simulink model "model"  (R2021a)
settings: Solver=ode4  StartTime=0.0  StopTime=sim_time  FixedStep=0.001  RelTol=1e-3
values from neighbouring files (symbols this model uses):
  ABS_ON = 0    [initialization.m]    (also in result_analysis.m = 1)
  Af = 2.36    [initialization.m]
  battery_capacity = 58*3.6*10^6    (= 208800000)    [initialization.m]
  battery_limit = 99    [initialization.m]
  brake_start = 10    [initialization.m]    (also in result_analysis.m)
  brakes = 1    [initialization.m]    (also in result_analysis.m)
  Cm = 310    [initialization.m]
  Cx = 0.27    [initialization.m]
  EBD_ON = 0    [initialization.m]    (also in result_analysis.m = 1)
  eta = 0.90    (= 0.9)    [initialization.m]
  Fx_lim = m*30    (= 54360)    [initialization.m]
  Fz = m*g/2    (= 8887.86)    [initialization.m]
  Gr = 10.5    [initialization.m]
  h = 0.55    [initialization.m]
  Ir = 1    [initialization.m]
  L = 2.77    [initialization.m]
  m = 1812    [initialization.m]
  mu = 0.5    [initialization.m]    (also in result_analysis.m)
  Pacn = Pace'    [initialization.m]
  pedal = 1    [initialization.m]    (also in result_analysis.m)
  phi = 0.95    [initialization.m]
  Pmax = 150000    [initialization.m]
  R = (D+2*H)/(2*1000)    (= 0.3488)    [initialization.m]
  regTorque = -0.1*g*R*m/(Gr)    (= -59.0492489143)    [initialization.m]
  rho = 1.225    [initialization.m]
  sim_time = 50    [initialization.m]    (also in result_analysis.m = 30)
  TCS_ON = 1    [initialization.m]    (also in result_analysis.m = 0)
  velstart = 0.5    [initialization.m]    (also in result_analysis.m = 30)
libraries: pid_lib x4
(part 1 of 2)
settings Model: Creator=Utente  LastModifiedBy=Utente
settings DataIOCC: ReturnWorkspaceOutputs=off

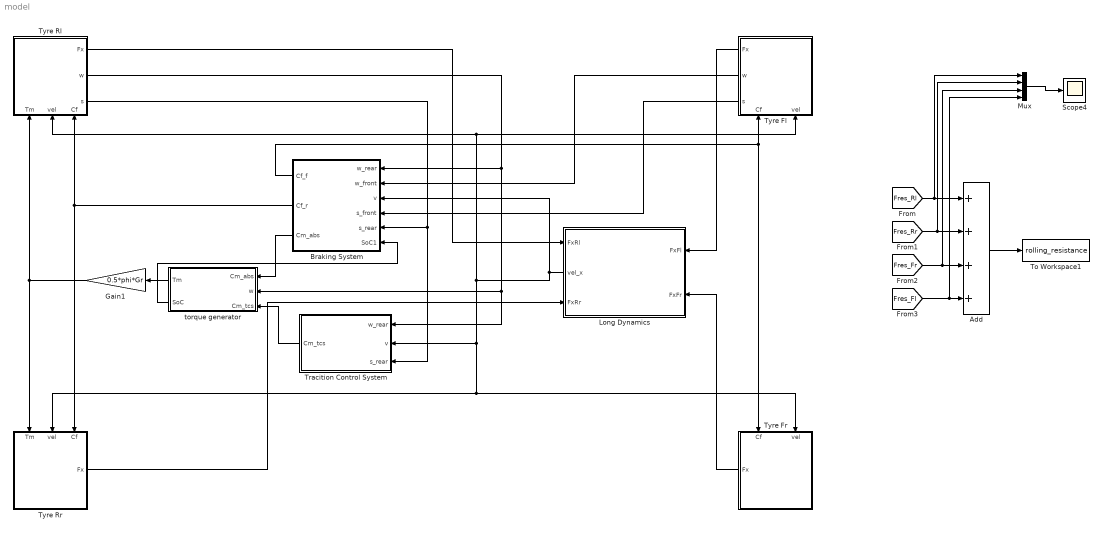
== system model ==
  Add : Sum  Inputs=++++
  Braking System : Subsystem
  Gain1 : Gain  Gain=0.5*phi*Gr
  Long Dynamics : Subsystem
      settings: PortSchema="{\"entries\":[{\"content\":{\"sides\":[{\"content\":{\"connectorIds\":[\"In1\",\"Out1\",\"In2\"]},\"type\":\"ConnectorPlacement.EquallySpacedRectSide\",\"uuid\":\"f4bfbc8e-e09b-460b-b847-06647d23fd6c\"},{\"content\":{\"connectorIds\":[\"In3\",\"In4\"],\"side\":\"RIGHT\"},\"type\":\"ConnectorPlacement.EquallySpacedRectSide\",\"uuid\":\"843119d8-e9e9-4b71-b659-44edd5e92d7e\"},{\"content\":{\"connectorIds\":[],\"side\":\"TOP\"},\"type\":\"ConnectorPlacement.EquallySpacedRectSide\",\"uuid\":\"d54a9cef-2e9c-4051-86e0-74dc12721ec3\"}]},\"type\":\"ConnectorPlacement.EquallySpacedConnector\",\"uuid\":\"90a496b7-624e-4a31-ae84-9184d6a3237c\"}],\"packageUris\":[\"http://schema.mathworks.com/mf0/Connector/R2020b\"],\"version\":\"1.0\"}"
  Mux : Mux
  Scope4 : Scope
  To Workspace1 : ToWorkspace  VariableName=rolling_resistance  SampleTime=-1
  Tracition Control System : Subsystem
  Tyre Fl : Subsystem
      settings: PortSchema="{\"entries\":[{\"content\":{\"sides\":[{\"content\":{\"connectorIds\":[]},\"type\":\"ConnectorPlacement.EquallySpacedRectSide\",\"uuid\":\"645908f1-aef9-45cd-aa2f-84533f90cce5\"},{\"content\":{\"connectorIds\":[\"Out1\",\"Out2\",\"Out3\"],\"side\":\"RIGHT\"},\"type\":\"ConnectorPlacement.EquallySpacedRectSide\",\"uuid\":\"ac122367-fdda-410e-89ff-4b44cb142215\"},{\"content\":{\"connectorIds\":[],\"side\":\"TOP\"},\"type\":\"ConnectorPlacement.EquallySpacedRectSide\",\"uuid\":\"c31bcef3-36ae-47f3-b214-8c835aef2e2f\"},{\"content\":{\"connectorIds\":[\"In1\",\"In2\"],\"side\":\"BOTTOM\"},\"type\":\"ConnectorPlacement.EquallySpacedRectSide\",\"uuid\":\"9005a4b9-f595-4b37-a59c-f0ffecb85b0d\"}]},\"type\":\"ConnectorPlacement.EquallySpacedConnector\",\"uuid\":\"352140d8-d969-4d1c-ae25-dc72e5f25954\"}],\"packageUris\":[\"http://schema.mathworks.com/mf0/Connector/R2020b\"],\"version\":\"1.0\"}"
  Tyre Fr : Subsystem
      settings: PortSchema="{\"entries\":[{\"content\":{\"sides\":[{\"content\":{\"connectorIds\":[]},\"type\":\"ConnectorPlacement.EquallySpacedRectSide\",\"uuid\":\"645908f1-aef9-45cd-aa2f-84533f90cce5\"},{\"content\":{\"connectorIds\":[\"Out1\"],\"side\":\"RIGHT\"},\"type\":\"ConnectorPlacement.EquallySpacedRectSide\",\"uuid\":\"ac122367-fdda-410e-89ff-4b44cb142215\"},{\"content\":{\"connectorIds\":[],\"side\":\"TOP\"},\"type\":\"ConnectorPlacement.EquallySpacedRectSide\",\"uuid\":\"c31bcef3-36ae-47f3-b214-8c835aef2e2f\"},{\"content\":{\"connectorIds\":[\"In1\",\"In2\"],\"side\":\"BOTTOM\"},\"type\":\"ConnectorPlacement.EquallySpacedRectSide\",\"uuid\":\"9005a4b9-f595-4b37-a59c-f0ffecb85b0d\"}]},\"type\":\"ConnectorPlacement.EquallySpacedConnector\",\"uuid\":\"352140d8-d969-4d1c-ae25-dc72e5f25954\"}],\"packageUris\":[\"http://schema.mathworks.com/mf0/Connector/R2020b\"],\"version\":\"1.0\"}"
  Tyre Rl : Subsystem
      settings: PortSchema="{\"entries\":[{\"content\":{\"sides\":[{\"content\":{\"connectorIds\":[]},\"type\":\"ConnectorPlacement.EquallySpacedRectSide\",\"uuid\":\"645908f1-aef9-45cd-aa2f-84533f90cce5\"},{\"content\":{\"connectorIds\":[\"Out1\",\"Out2\",\"Out3\"],\"side\":\"RIGHT\"},\"type\":\"ConnectorPlacement.EquallySpacedRectSide\",\"uuid\":\"ac122367-fdda-410e-89ff-4b44cb142215\"},{\"content\":{\"connectorIds\":[],\"side\":\"TOP\"},\"type\":\"ConnectorPlacement.EquallySpacedRectSide\",\"uuid\":\"c31bcef3-36ae-47f3-b214-8c835aef2e2f\"},{\"content\":{\"connectorIds\":[\"In1\",\"In2\",\"In3\"],\"side\":\"BOTTOM\"},\"type\":\"ConnectorPlacement.EquallySpacedRectSide\",\"uuid\":\"9005a4b9-f595-4b37-a59c-f0ffecb85b0d\"}]},\"type\":\"ConnectorPlacement.EquallySpacedConnector\",\"uuid\":\"352140d8-d969-4d1c-ae25-dc72e5f25954\"}],\"packageUris\":[\"http://schema.mathworks.com/mf0/Connector/R2020b\"],\"version\":\"1.0\"}"
  Tyre Rr : Subsystem
      settings: PortSchema="{\"entries\":[{\"content\":{\"sides\":[{\"content\":{\"connectorIds\":[]},\"type\":\"ConnectorPlacement.EquallySpacedRectSide\",\"uuid\":\"645908f1-aef9-45cd-aa2f-84533f90cce5\"},{\"content\":{\"connectorIds\":[\"Out1\"],\"side\":\"RIGHT\"},\"type\":\"ConnectorPlacement.EquallySpacedRectSide\",\"uuid\":\"ac122367-fdda-410e-89ff-4b44cb142215\"},{\"content\":{\"connectorIds\":[],\"side\":\"TOP\"},\"type\":\"ConnectorPlacement.EquallySpacedRectSide\",\"uuid\":\"c31bcef3-36ae-47f3-b214-8c835aef2e2f\"},{\"content\":{\"connectorIds\":[\"In1\",\"In2\",\"In3\"],\"side\":\"BOTTOM\"},\"type\":\"ConnectorPlacement.EquallySpacedRectSide\",\"uuid\":\"9005a4b9-f595-4b37-a59c-f0ffecb85b0d\"}]},\"type\":\"ConnectorPlacement.EquallySpacedConnector\",\"uuid\":\"352140d8-d969-4d1c-ae25-dc72e5f25954\"}],\"packageUris\":[\"http://schema.mathworks.com/mf0/Connector/R2020b\"],\"version\":\"1.0\"}"
  torque generator : Subsystem
      settings: PortSchema="{\"entries\":[{\"content\":{\"sides\":[{\"content\":{\"connectorIds\":[\"Out1\",\"Out2\"]},\"type\":\"ConnectorPlacement.EquallySpacedRectSide\",\"uuid\":\"aba36ed2-9b43-4b5e-a032-9d2e14e4331b\"},{\"content\":{\"connectorIds\":[\"In1\",\"In2\",\"In3\"],\"side\":\"RIGHT\"},\"type\":\"ConnectorPlacement.EquallySpacedRectSide\",\"uuid\":\"b07ddcf2-8a87-4222-b0b4-5c7ab20df70e\"},{\"content\":{\"connectorIds\":[],\"side\":\"TOP\"},\"type\":\"ConnectorPlacement.EquallySpacedRectSide\",\"uuid\":\"d129fe33-93da-4841-be61-7298d53a860e\"}]},\"type\":\"ConnectorPlacement.EquallySpacedConnector\",\"uuid\":\"86c7d2c9-2449-4d03-9cdc-c51b2e17982e\"}],\"packageUris\":[\"http://schema.mathworks.com/mf0/Connector/R2020b\"],\"version\":\"1.0\"}"
  wires:
  Tyre Rl/1(Fx) -> Long Dynamics/1(FxRl)
  Tyre Rr/1(Fx) -> Long Dynamics/2(FxRr)
  Tyre Fl/1(Fx) -> Long Dynamics/3(FxFl)
  Tyre Fr/1(Fx) -> Long Dynamics/4(FxFr)
  Tyre Fl/2(w) -> Braking System/2(w_front)
  Tyre Rl/3(s) -> Tracition Control System/3(s_rear), Braking System/5(s_rear)
  Tyre Fl/3(s) -> Braking System/4(s_front)
  Braking System/1(Cf_f) -> Tyre Fr/2(Cf), Tyre Fl/2(Cf)
  Gain1/1 -> Tyre Rl/1(Tm), Tyre Rr/1(Tm)
  Long Dynamics/1(vel_x) -> Tyre Rl/2(vel), Tyre Fl/1(vel), Tracition Control System/2(v), Tyre Rr/2(vel), Tyre Fr/1(vel), Braking System/3(v)
  [Fres_Rl] -> Mux/1, Add/1
  [Fres_Rr] -> Mux/2, Add/2
  [Fres_Fr] -> Mux/3, Add/3
  [Fres_Fl] -> Mux/4, Add/4
  Add/1 -> To Workspace1/1
  Mux/1 -> Scope4/1
  Tyre Rl/2(w) -> Tracition Control System/1(w_rear), torque generator/2(w), Braking System/1(w_rear)
  Braking System/2(Cf_r) -> Tyre Rl/3(Cf), Tyre Rr/3(Cf)
  Braking System/3(Cm_abs) -> torque generator/1(Cm_abs)
  Tracition Control System/1(Cm_tcs) -> torque generator/3(Cm_tcs)
  torque generator/1(Tm) -> Gain1/1
  torque generator/2(SoC) -> Braking System/6(SoC1)

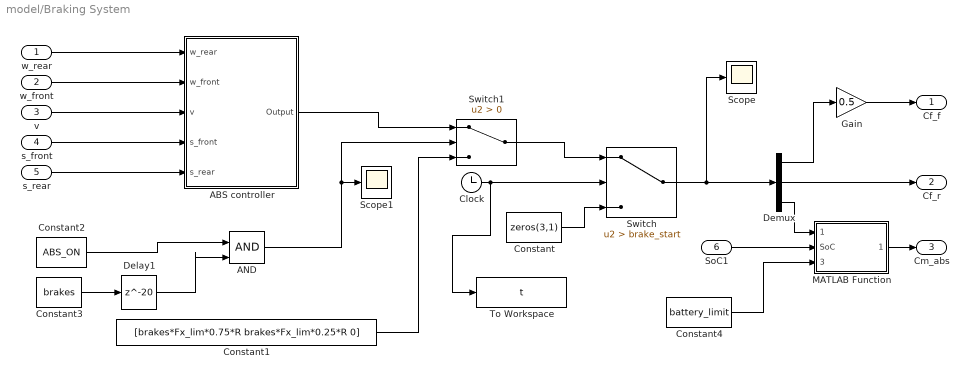
== system model/Braking System ==
  w_rear : Inport
  w_front : Inport  Port=2
  v : Inport  Port=3
  s_front : Inport  Port=4
  s_rear : Inport  Port=5
  SoC1 : Inport  Port=6
  ABS controller : Subsystem
  AND : Logic  IconShape=distinctive  AllPortsSameDT=off  OutDataTypeStr=boolean
  Clock : Clock
  Constant : Constant  Value=zeros(3,1)
  Constant1 : Constant  Value=[brakes*Fx_lim*0.75*R brakes*Fx_lim*0.25*R 0]
  Constant2 : Constant  Value=ABS_ON
  Constant3 : Constant  Value=brakes
  Constant4 : Constant  Value=battery_limit
  Delay1 : Delay  DelayLength=20
  Demux : Demux  Outputs=3
  Gain : Gain  Gain=0.5
  MATLAB Function : MATLAB Function  TreatAsAtomicUnit=on
  Scope : Scope
  Scope1 : Scope
  Switch : Switch  Criteria=u2 > Threshold  Threshold=brake_start
  Switch1 : Switch  Criteria=u2 > Threshold
  To Workspace : ToWorkspace  VariableName=t  SampleTime=-1
  Cf_f : Outport
  Cf_r : Outport  Port=2
  Cm_abs : Outport  Port=3
  wires:
  Constant/1 -> Switch/3
  Demux/1 -> Gain/1
  w_rear/1 -> ABS controller/1(w_rear)
  w_front/1 -> ABS controller/2(w_front)
  v/1 -> ABS controller/3(v)
  s_front/1 -> ABS controller/4(s_front)
  s_rear/1 -> ABS controller/5(s_rear)
  Switch1/1 -> Switch/1
  ABS controller/1(Output) -> Switch1/1
  Constant2/1 -> AND/1
  AND/1 -> Switch1/2, Scope1/1
  Constant3/1 -> Delay1/1
  Constant1/1 -> Switch1/3
  Switch/1 -> Demux/1, Scope/1
  Demux/3 -> MATLAB Function/1(Cm_abs_in)
  Clock/1 -> Switch/2, To Workspace/1
  Demux/2 -> Cf_r/1
  Gain/1 -> Cf_f/1
  Delay1/1 -> AND/2
  Constant4/1 -> MATLAB Function/3(battery_limit)
  SoC1/1 -> MATLAB Function/2(SoC)
  MATLAB Function/1(Cm_abs_out) -> Cm_abs/1

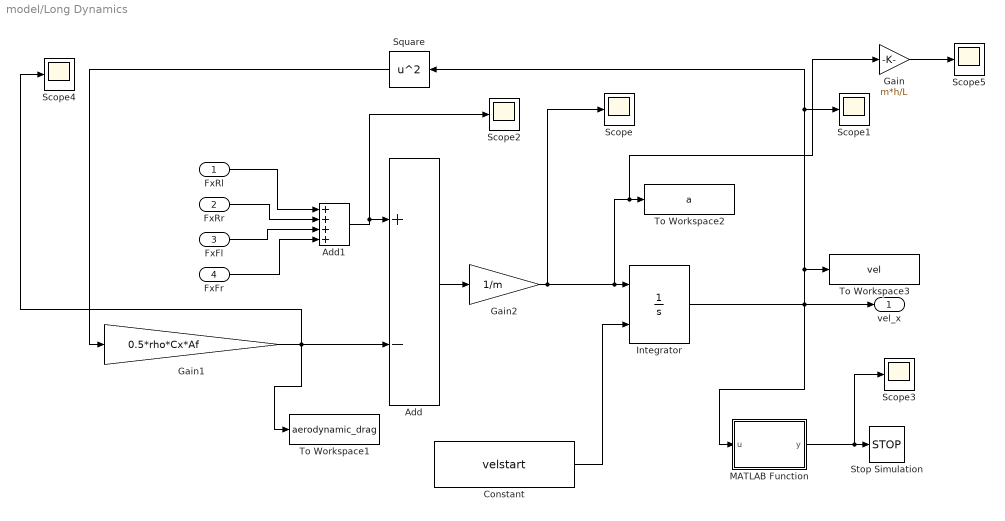
== system model/Long Dynamics ==
  FxRl : Inport
  FxRr : Inport  Port=2
  FxFl : Inport  Port=3
  FxFr : Inport  Port=4
  Add : Sum  Inputs=+-
  Add1 : Sum  Inputs=++++
  Constant : Constant  Value=velstart
  Gain : Gain  Gain=m*h/L
  Gain1 : Gain  Gain=0.5*rho*Cx*Af
  Gain2 : Gain  Gain=1/m
  Integrator : Integrator  InitialConditionSource=external  LimitOutput=on  LowerSaturationLimit=0
  MATLAB Function : MATLAB Function  TreatAsAtomicUnit=on
  Scope{,1..5} (6 alike) : Scope
  Square : Math  Operator=square  SaturateOnIntegerOverflow=on
  Stop Simulation : Stop
  To Workspace1 : ToWorkspace  VariableName=aerodynamic_drag  SampleTime=-1
  To Workspace2 : ToWorkspace  VariableName=a  SampleTime=-1
  To Workspace3 : ToWorkspace  VariableName=vel  SampleTime=-1
  vel_x : Outport
  wires:
  Add/1 -> Gain2/1
  Square/1 -> Gain1/1
  Constant/1 -> Integrator/2
  FxRl/1 -> Add1/1
  Gain1/1 -> To Workspace1/1, Scope4/1, Add/2
  Gain2/1 -> Gain/1, To Workspace2/1, Integrator/1, Scope/1
  FxRr/1 -> Add1/2
  FxFl/1 -> Add1/3
  FxFr/1 -> Add1/4
  Integrator/1 -> MATLAB Function/1(u), vel_x/1, To Workspace3/1, Square/1, Scope1/1
  MATLAB Function/1(y) -> Scope3/1, Stop Simulation/1
  Add1/1 -> Scope2/1, Add/1
  Gain/1 -> Scope5/1

== system model/Tracition Control System ==
  w_rear : Inport
  v : Inport  Port=2
  s_rear : Inport  Port=3
  AND : Logic  IconShape=distinctive  AllPortsSameDT=off  OutDataTypeStr=boolean
  Clock : Clock
  Constant : Constant  Value=0
  Constant2 : Constant  Value=regTorque*0.5*phi*Gr
  Constant3 : Constant  Value=TCS_ON
  Constant4 : Constant  Value=pedal
  Delay : Delay  DelayLength=20
  Scope : Scope
  Scope1 : Scope
  Switch : Switch  Criteria=u2 > Threshold  Threshold=sim_time
  Switch1 : Switch  Criteria=u2 > Threshold
  TCS controller : Subsystem
  Cm_tcs : Outport
  wires:
  Constant/1 -> Switch1/3
  Clock/1 -> Switch/2
  w_rear/1 -> TCS controller/1(w_rear)
  v/1 -> TCS controller/2(v)
  s_rear/1 -> TCS controller/3(s_rear)
  TCS controller/1(Output) -> Switch1/1
  AND/1 -> Switch1/2, Scope1/1
  Switch1/1 -> Switch/3
  Constant2/1 -> Switch/1
  Constant3/1 -> AND/1
  Switch/1 -> Cm_tcs/1, Scope/1
  Constant4/1 -> Delay/1
  Delay/1 -> AND/2

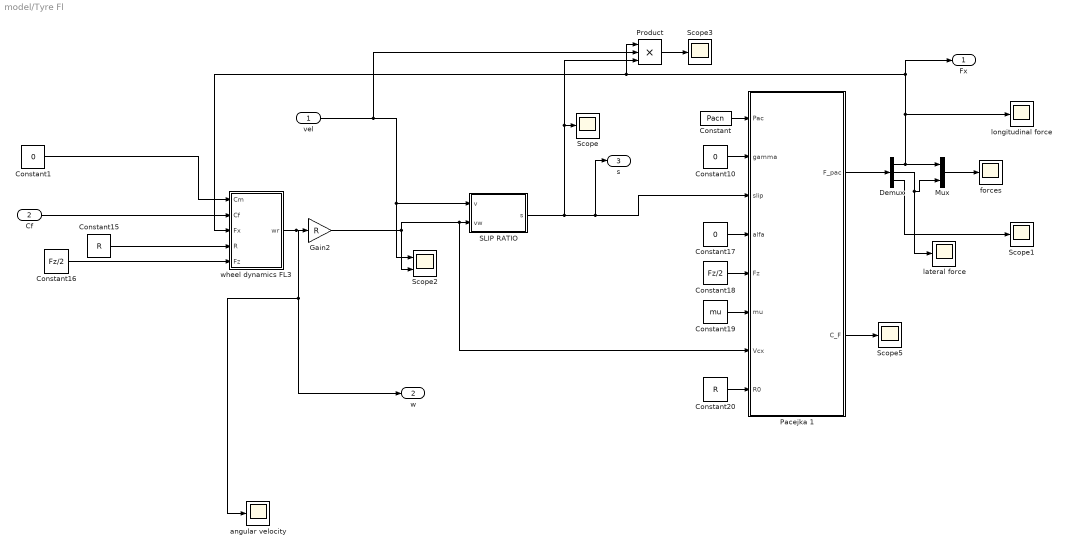
== system model/Tyre Fl ==
  vel : Inport
  Cf : Inport  Port=2
  Constant : Constant  Value=Pacn
  Constant1 : Constant  Value=0
  Constant10 : Constant  Value=0
  Constant15 : Constant  Value=R
  Constant16 : Constant  Value=Fz/2
  Constant17 : Constant  Value=0
  Constant18 : Constant  Value=Fz/2
  Constant19 : Constant  Value=mu
  Constant20 : Constant  Value=R
  Demux : Demux  Outputs=3
  Gain2 : Gain  Gain=R
  Mux : Mux  Inputs=2
  Pacejka 1 : MATLAB Function  TreatAsAtomicUnit=on
  Product : Product  Inputs=3
  SLIP RATIO : MATLAB Function  TreatAsAtomicUnit=on
  Scope{,1,3,5} (4 alike) : Scope
  Scope2 : Scope  NumInputPorts=2
  angular velocity : Scope
  forces : Scope
  lateral force : Scope
  longitudinal force : Scope
  wheel dynamics FL3 : Subsystem
  Fx : Outport
  w : Outport  Port=2
  s : Outport  Port=3
  wires:
  Constant19/1 -> Pacejka 1/6(mu)
  Constant17/1 -> Pacejka 1/4(alfa)
  Pacejka 1/2(C_F) -> Scope5/1
  Constant20/1 -> Pacejka 1/8(R0)
  Constant15/1 -> wheel dynamics FL3/4(R)
  Constant1/1 -> wheel dynamics FL3/1(Cm)
  wheel dynamics FL3/1(wr) -> w/1, angular velocity/1, Gain2/1
  Constant18/1 -> Pacejka 1/5(Fz)
  Constant16/1 -> wheel dynamics FL3/5(Fz)
  Demux/1 -> Fx/1, Product/1, wheel dynamics FL3/3(Fx), longitudinal force/1, Mux/1
  Mux/1 -> forces/1
  Pacejka 1/1(F_pac) -> Demux/1
  Demux/2 -> Mux/2, lateral force/1
  Constant/1 -> Pacejka 1/1(Pac)
  Constant10/1 -> Pacejka 1/2(gamma)
  Gain2/1 -> Scope2/2, Pacejka 1/7(Vcx), SLIP RATIO/2(vw)
  Demux/3 -> Scope1/1
  vel/1 -> Product/2, Scope2/1, SLIP RATIO/1(v)
  SLIP RATIO/1(s) -> Product/3, Scope/1, s/1, Pacejka 1/3(slip)
  Cf/1 -> wheel dynamics FL3/2(Cf)
  Product/1 -> Scope3/1

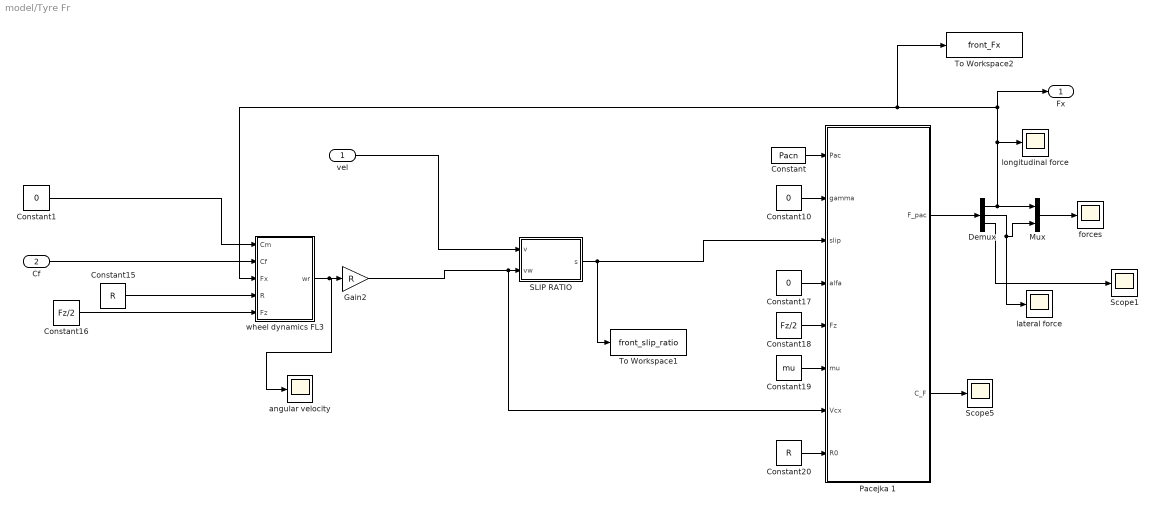
== system model/Tyre Fr ==
  vel : Inport
  Cf : Inport  Port=2
  Constant : Constant  Value=Pacn
  Constant1 : Constant  Value=0
  Constant10 : Constant  Value=0
  Constant15 : Constant  Value=R
  Constant16 : Constant  Value=Fz/2
  Constant17 : Constant  Value=0
  Constant18 : Constant  Value=Fz/2
  Constant19 : Constant  Value=mu
  Constant20 : Constant  Value=R
  Demux : Demux  Outputs=3
  Gain2 : Gain  Gain=R
  Mux : Mux  Inputs=2
  Pacejka 1 : MATLAB Function  TreatAsAtomicUnit=on
  SLIP RATIO : MATLAB Function  TreatAsAtomicUnit=on
  Scope1 : Scope
  Scope5 : Scope
  To Workspace1 : ToWorkspace  VariableName=front_slip_ratio  SampleTime=-1
  To Workspace2 : ToWorkspace  VariableName=front_Fx  SampleTime=-1
  angular velocity : Scope
  forces : Scope
  lateral force : Scope
  longitudinal force : Scope
  wheel dynamics FL3 : Subsystem
  Fx : Outport
  wires:
  Constant19/1 -> Pacejka 1/6(mu)
  Constant17/1 -> Pacejka 1/4(alfa)
  Pacejka 1/2(C_F) -> Scope5/1
  Constant20/1 -> Pacejka 1/8(R0)
  Constant15/1 -> wheel dynamics FL3/4(R)
  Constant1/1 -> wheel dynamics FL3/1(Cm)
  wheel dynamics FL3/1(wr) -> angular velocity/1, Gain2/1
  Constant18/1 -> Pacejka 1/5(Fz)
  Constant16/1 -> wheel dynamics FL3/5(Fz)
  Demux/1 -> Fx/1, To Workspace2/1, wheel dynamics FL3/3(Fx), longitudinal force/1, Mux/1
  Mux/1 -> forces/1
  Pacejka 1/1(F_pac) -> Demux/1
  Demux/2 -> Mux/2, lateral force/1
  Constant/1 -> Pacejka 1/1(Pac)
  Constant10/1 -> Pacejka 1/2(gamma)
  Gain2/1 -> Pacejka 1/7(Vcx), SLIP RATIO/2(vw)
  Demux/3 -> Scope1/1
  vel/1 -> SLIP RATIO/1(v)
  SLIP RATIO/1(s) -> To Workspace1/1, Pacejka 1/3(slip)
  Cf/1 -> wheel dynamics FL3/2(Cf)

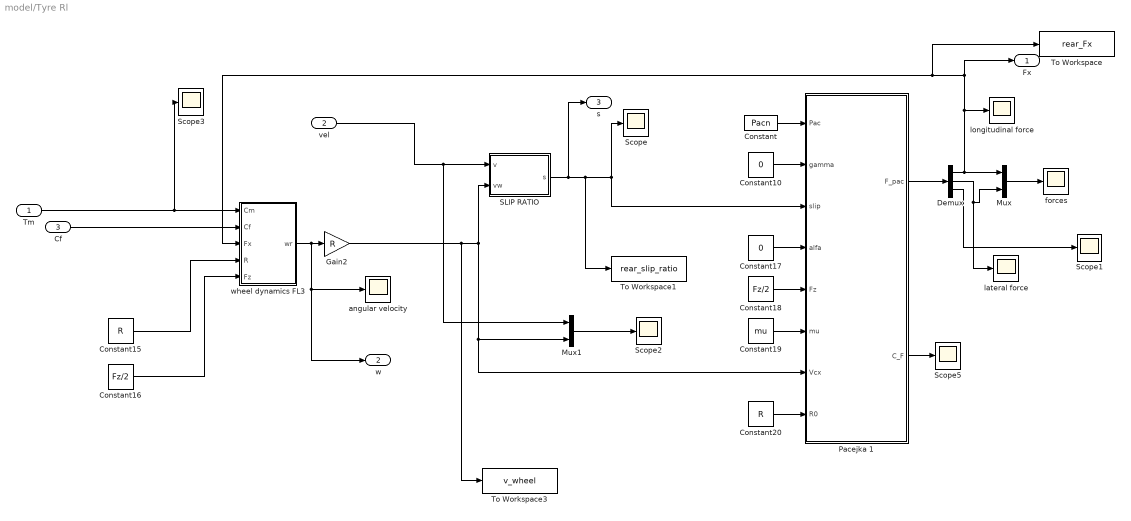
== system model/Tyre Rl ==
  Tm : Inport
  vel : Inport  Port=2
  Cf : Inport  Port=3
  Constant : Constant  Value=Pacn
  Constant10 : Constant  Value=0
  Constant15 : Constant  Value=R
  Constant16 : Constant  Value=Fz/2
  Constant17 : Constant  Value=0
  Constant18 : Constant  Value=Fz/2
  Constant19 : Constant  Value=mu
  Constant20 : Constant  Value=R
  Demux : Demux  Outputs=3
  Gain2 : Gain  Gain=R
  Mux : Mux  Inputs=2
  Mux1 : Mux  Inputs=2
  Pacejka 1 : MATLAB Function  TreatAsAtomicUnit=on
  SLIP RATIO : MATLAB Function  TreatAsAtomicUnit=on
  Scope{,1..3,5} (5 alike) : Scope
  To Workspace : ToWorkspace  VariableName=rear_Fx  SampleTime=-1
  To Workspace1 : ToWorkspace  VariableName=rear_slip_ratio  SampleTime=-1
  To Workspace3 : ToWorkspace  VariableName=v_wheel  SampleTime=-1
  angular velocity : Scope
  forces : Scope
  lateral force : Scope
  longitudinal force : Scope
  wheel dynamics FL3 : Subsystem
  Fx : Outport
  w : Outport  Port=2
  s : Outport  Port=3
  wires:
  Constant19/1 -> Pacejka 1/6(mu)
  Constant17/1 -> Pacejka 1/4(alfa)
  Pacejka 1/2(C_F) -> Scope5/1
  Constant20/1 -> Pacejka 1/8(R0)
  Constant15/1 -> wheel dynamics FL3/4(R)
  Tm/1 -> Scope3/1, wheel dynamics FL3/1(Cm)
  wheel dynamics FL3/1(wr) -> angular velocity/1, w/1, Gain2/1
  Constant18/1 -> Pacejka 1/5(Fz)
  Constant16/1 -> wheel dynamics FL3/5(Fz)
  Demux/1 -> Fx/1, To Workspace/1, wheel dynamics FL3/3(Fx), longitudinal force/1, Mux/1
  Mux/1 -> forces/1
  Pacejka 1/1(F_pac) -> Demux/1
  Demux/2 -> Mux/2, lateral force/1
  Constant/1 -> Pacejka 1/1(Pac)
  Constant10/1 -> Pacejka 1/2(gamma)
  Demux/3 -> Scope1/1
  Gain2/1 -> To Workspace3/1, Mux1/2, Pacejka 1/7(Vcx), SLIP RATIO/2(vw)
  vel/1 -> SLIP RATIO/1(v), Mux1/1
  SLIP RATIO/1(s) -> s/1, To Workspace1/1, Scope/1, Pacejka 1/3(slip)
  Mux1/1 -> Scope2/1
  Cf/1 -> wheel dynamics FL3/2(Cf)

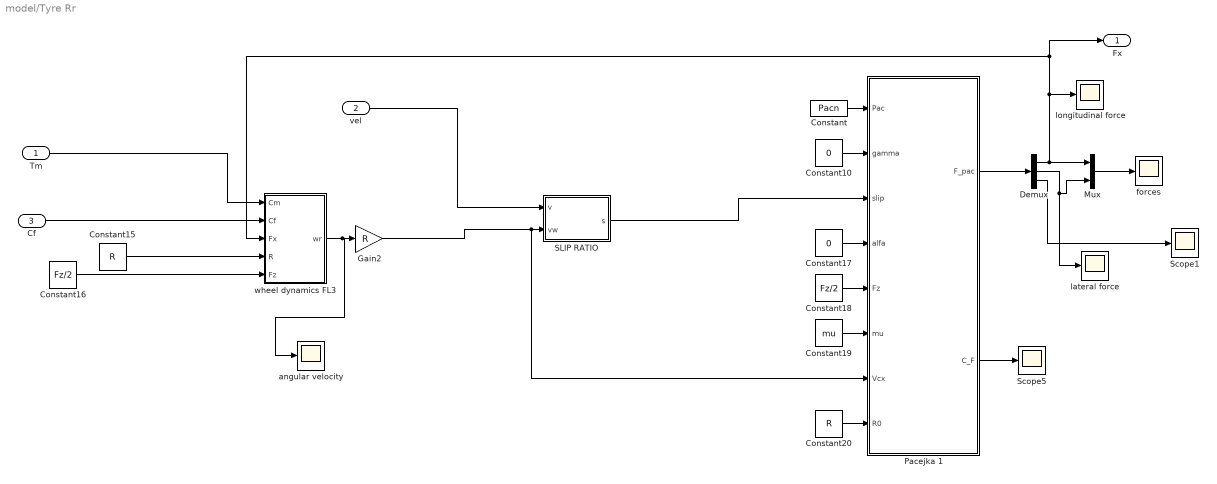
== system model/Tyre Rr ==
  Tm : Inport
  vel : Inport  Port=2
  Cf : Inport  Port=3
  Constant : Constant  Value=Pacn
  Constant10 : Constant  Value=0
  Constant15 : Constant  Value=R
  Constant16 : Constant  Value=Fz/2
  Constant17 : Constant  Value=0
  Constant18 : Constant  Value=Fz/2
  Constant19 : Constant  Value=mu
  Constant20 : Constant  Value=R
  Demux : Demux  Outputs=3
  Gain2 : Gain  Gain=R
  Mux : Mux  Inputs=2
  Pacejka 1 : MATLAB Function  TreatAsAtomicUnit=on
  SLIP RATIO : MATLAB Function  TreatAsAtomicUnit=on
  Scope1 : Scope
  Scope5 : Scope
  angular velocity : Scope
  forces : Scope
  lateral force : Scope
  longitudinal force : Scope
  wheel dynamics FL3 : Subsystem
  Fx : Outport
  wires:
  Constant19/1 -> Pacejka 1/6(mu)
  Constant17/1 -> Pacejka 1/4(alfa)
  Pacejka 1/2(C_F) -> Scope5/1
  Constant20/1 -> Pacejka 1/8(R0)
  Constant15/1 -> wheel dynamics FL3/4(R)
  Tm/1 -> wheel dynamics FL3/1(Cm)
  Constant18/1 -> Pacejka 1/5(Fz)
  Constant16/1 -> wheel dynamics FL3/5(Fz)
  Demux/1 -> Fx/1, wheel dynamics FL3/3(Fx), longitudinal force/1, Mux/1
  Mux/1 -> forces/1
  Pacejka 1/1(F_pac) -> Demux/1
  Demux/2 -> Mux/2, lateral force/1
  Constant/1 -> Pacejka 1/1(Pac)
  Constant10/1 -> Pacejka 1/2(gamma)
  Gain2/1 -> Pacejka 1/7(Vcx), SLIP RATIO/2(vw)
  Demux/3 -> Scope1/1
  vel/1 -> SLIP RATIO/1(v)
  SLIP RATIO/1(s) -> Pacejka 1/3(slip)
  Cf/1 -> wheel dynamics FL3/2(Cf)
  wheel dynamics FL3/1(wr) -> angular velocity/1, Gain2/1

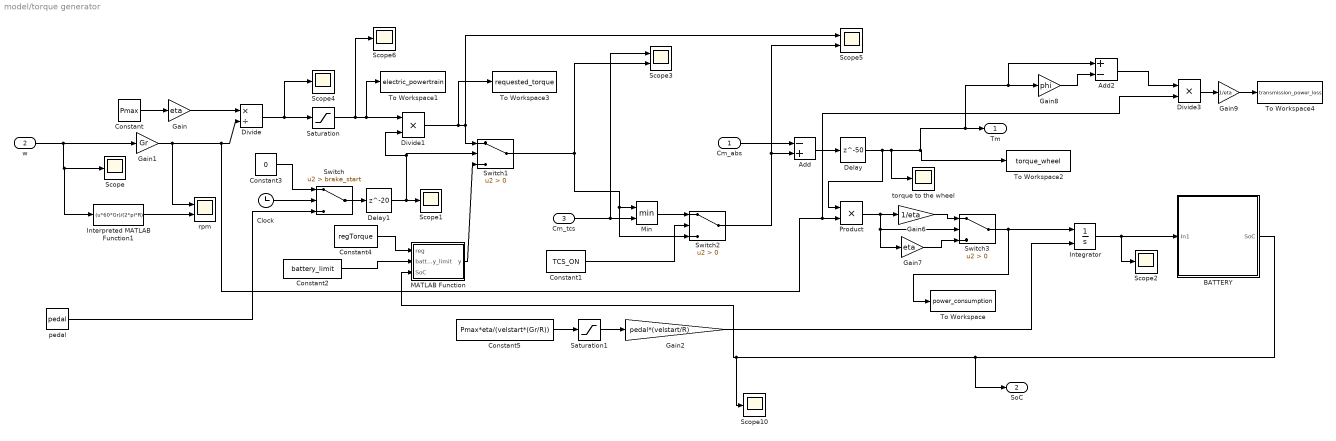
== system model/torque generator ==
  Cm_abs : Inport
  w : Inport  Port=2
  Cm_tcs : Inport  Port=3
  Add : Sum  Inputs=-+
  Add2 : Sum  Inputs=+-
  BATTERY : Subsystem
  Clock : Clock
  Constant : Constant  Value=Pmax
  Constant1 : Constant  Value=TCS_ON
  Constant2 : Constant  Value=battery_limit
  Constant3 : Constant  Value=0
  Constant4 : Constant  Value=regTorque
  Constant5 : Constant  Value=Pmax*eta/(velstart*(Gr/R))
  Delay : Delay  DelayLength=50
  Delay1 : Delay  DelayLength=20
  Divide : Product  Inputs=*/
  Divide1 : Product  Inputs=**
  Divide3 : Product
  Gain : Gain  Gain=eta
  Gain1 : Gain  Gain=Gr
  Gain2 : Gain  Gain=pedal*(velstart/R)
  Gain6 : Gain  Gain=1/eta
  Gain7 : Gain  Gain=eta
  Gain8 : Gain  Gain=phi
  Gain9 : Gain  Gain=1/eta
  Integrator : Integrator  InitialConditionSource=external
  Interpreted MATLAB Function1 : MATLABFcn  MATLABFcn=(u*60*Gr)/(2*pi*R)
  MATLAB Function : MATLAB Function  TreatAsAtomicUnit=on
  Min : MinMax  Inputs=2
  Product : Product
  Saturation : Saturate  UpperLimit=Cm  LowerLimit=0
  Saturation1 : Saturate  UpperLimit=Cm  LowerLimit=-Cm
  Scope{,1..2,4,6,10} (6 alike) : Scope
  Scope3 : Scope  NumInputPorts=2
  Scope5 : Scope  NumInputPorts=2
  Switch : Switch  Criteria=u2 > Threshold  Threshold=brake_start
  Switch1 : Switch  Criteria=u2 > Threshold
  Switch2 : Switch  Criteria=u2 > Threshold
  Switch3 : Switch  Criteria=u2 > Threshold
  To Workspace : ToWorkspace  VariableName=power_consumption  SampleTime=-1
  To Workspace1 : ToWorkspace  VariableName=electric_powertrain  SampleTime=-1
  To Workspace2 : ToWorkspace  VariableName=torque_wheel  SampleTime=-1
  To Workspace3 : ToWorkspace  VariableName=requested_torque  SampleTime=-1
  To Workspace4 : ToWorkspace  VariableName=transmission_power_loss  SampleTime=-1
  pedal : Constant  Value=pedal
  rpm : Scope  NumInputPorts=2
  torque to the wheel : Scope
  Tm : Outport
  SoC : Outport  Port=2
  wires:
  Constant/1 -> Gain/1
  Divide/1 -> Saturation/1, Scope4/1
  Saturation/1 -> Scope6/1, Divide1/1, To Workspace1/1
  Interpreted MATLAB Function1/1 -> rpm/2
  Gain/1 -> Divide/1
  Clock/1 -> Switch/2
  Constant3/1 -> Switch/1
  Divide1/1 -> To Workspace3/1, Scope5/1, Switch1/1
  Constant5/1 -> Saturation1/1
  Saturation1/1 -> Gain2/1
  Integrator/1 -> BATTERY/1(In1), Scope2/1
  Product/1 -> Switch3/2, Gain7/1, Gain6/1
  Gain2/1 -> Integrator/2
  Cm_tcs/1 -> Min/2, Scope3/1
  Constant1/1 -> Switch2/2
  Min/1 -> Switch2/1
  Add/1 -> Delay/1
  w/1 -> Gain1/1, Interpreted MATLAB Function1/1, Scope/1
  Switch1/1 -> Scope3/2, Switch2/3, Min/1
  Switch3/1 -> To Workspace/1, Integrator/1
  Gain6/1 -> Switch3/1
  Gain7/1 -> Switch3/3
  Switch/1 -> Delay1/1
  Switch2/1 -> Scope5/2, Add/2
  Delay1/1 -> Divide1/2, Switch1/2, Scope1/1
  Constant4/1 -> MATLAB Function/1(reg)
  BATTERY/1(SoC) -> SoC/1, MATLAB Function/3(SoC), Scope10/1
  Cm_abs/1 -> Add/1
  Constant2/1 -> MATLAB Function/2(battery_limit)
  pedal/1 -> Switch/3
  MATLAB Function/1(y) -> Switch1/3
  Divide3/1 -> Gain9/1
  Gain8/1 -> Add2/2
  Add2/1 -> Divide3/1
  Gain9/1 -> To Workspace4/1
  Delay/1 -> Product/1, torque to the wheel/1, Add2/1, Gain8/1, Tm/1, To Workspace2/1
  Gain1/1 -> Divide3/2, Product/2, Divide/2, rpm/1

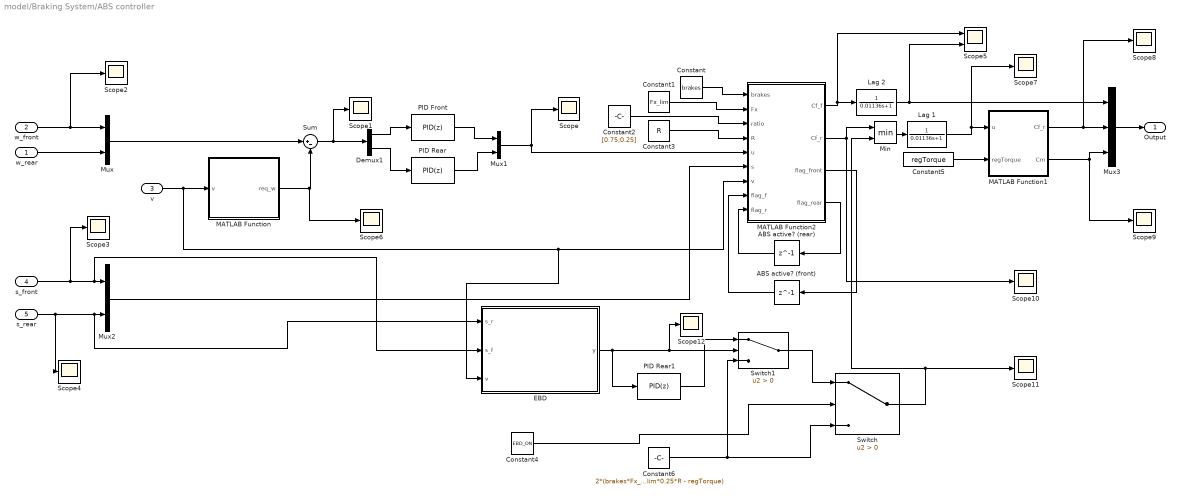
== system model/Braking System/ABS controller ==
  w_rear : Inport
  w_front : Inport  Port=2
  v : Inport  Port=3
  s_front : Inport  Port=4
  s_rear : Inport  Port=5
  " Lag 2" : TransferFcn  Denominator=[0.01136 1]
  ABS active? (front) : Delay  DelayLength=1
  ABS active? (rear) : Delay  DelayLength=1
  Constant : Constant  Value=brakes
  Constant1 : Constant  Value=Fx_lim
  Constant2 : Constant  Value=[0.75;0.25]
  Constant3 : Constant  Value=R
  Constant4 : Constant  Value=EBD_ON
  Constant5 : Constant  Value=regTorque
  Constant6 : Constant  Value=2*(brakes*Fx_lim*0.25*R - regTorque)
  Demux1 : Demux  Outputs=2
  EBD : MATLAB Function  TreatAsAtomicUnit=on
  Lag 1 : TransferFcn  Denominator=[0.01136 1]
  MATLAB Function : MATLAB Function  TreatAsAtomicUnit=on
  MATLAB Function1 : MATLAB Function  TreatAsAtomicUnit=on
  MATLAB Function2 : MATLAB Function  TreatAsAtomicUnit=on
  Min : MinMax  Inputs=2
  Mux : Mux  Inputs=2
  Mux1 : Mux  Inputs=2
  Mux2 : Mux  Inputs=2
  Mux3 : Mux  Inputs=3
  PID Front : pid_lib/PID Controller  Controller=PID  Form=Parallel  TimeDomain=Discrete-time  UseExternalTs=off  SampleTime=-1  IntegratorMethod=Forward Euler  FilterMethod=Forward Euler  ControllerParametersSource=internal  P=30  I=1.35  D=1  UseFilter=on  N=100  TunerSelectOption=Transfer Function Based (PID Tuner App)  InitialConditionSource=internal  InitialConditionForIntegrator=0  InitialConditionForFilter=0  DifferentiatorICPrevScaledInput=0  ExternalReset=none  TrackingMode=off  Kt=1  LimitOutput=on  SatLimitsSource=internal  UpperSaturationLimit=brakes*Fx_lim*0.75*R  LowerSaturationLimit=0  LinearizeAsGain=on  AntiWindupMode=none  Kb=1  POutMin=[]  POutMax=[]  IOutMin=[]  IOutMax=[]  DOutMin=[]  DOutMax=[]  NOutMin=[]  NOutMax=[]  SumOutMin=[]  SumOutMax=[]  SaturationOutMin=[]  SaturationOutMax=[]  PParamMin=[]  PParamMax=[]  IParamMin=[]  IParamMax=[]  DParamMin=[]  DParamMax=[]  NParamMin=[]  NParamMax=[]  KbParamMin=[]  KbParamMax=[]  KtParamMin=[]  KtParamMax=[]  KbOutMin=[]  KbOutMax=[]  KtOutMin=[]  KtOutMax=[]  IntegratorOutMin=[]  IntegratorOutMax=[]  FilterOutMin=[]  FilterOutMax=[]  SumI1OutMin=[]  SumI1OutMax=[]  SumI2OutMin=[]  SumI2OutMax=[]  SumI3OutMin=[]  SumI3OutMax=[]  SumI4OutMin=[]  SumI4OutMax=[]  SumDOutMin=[]  SumDOutMax=[]  DifferentiatorOutMin=[]  DifferentiatorOutMax=[]  FilterDiffOutCoefMin=[]  FilterDiffOutCoefMax=[]  ReciprocalOutMin=[]  ReciprocalOutMax=[]  SumDenOutMin=[]  SumDenOutMax=[]  SumNumOutMin=[]  SumNumOutMax=[]  DivideOutMin=[]  DivideOutMax=[]  UdiffTsProdOutMin=[]  UdiffTsProdOutMax=[]  NTsProdOutMin=[]  NTsProdOutMax=[]  UintegralTsProdOutMin=[]  UintegralTsProdOutMax=[]  UngainTsProdOutMin=[]  UngainTsProdOutMax=[]  IntegratorContinuousStateAttributes=''  IntegratorStateMustResolveToSignalObject=off  IntegratorRTWStateStorageClass=Auto  FilterContinuousStateAttributes=''  FilterStateMustResolveToSignalObject=off  FilterRTWStateStorageClass=Auto  ParallelPVariant=InternalParameters  IdealPVariant=Disabled  IVariant=InternalParameters  DVariant=InternalParameters  IntegratorVariant=Discrete  SatVariant=Enabled  AWVariant=Passthrough  PCopyVariant=Disabled  TRVariant=Disabled  FdbkBlocksVariant=Forward  IdealPFdbkVariant=Disabled  SatFdbkVariant=Disabled  DerivativeFilterVariant=ForwardEulerFilter  NVariant=InternalParameters  NCopyVariant=Disabled  FilterICVariant=InternalICsFilter  IntegratorICVariant=InternalICs  ExternalResetVariant=Disabled  TRSumVariant=Passthrough  SumFdbkVariant=Disabled  SumVariant=Sum_PID  TsampFilterVariant=InternalTs  TsampNgainVariant=Passthrough  TsampIntegralVariant=Passthrough  ExternalSaturationOutDataTypeStr=Inherit: Same as second input
  PID Rear : pid_lib/PID Controller  Controller=PID  Form=Parallel  TimeDomain=Discrete-time  UseExternalTs=off  SampleTime=-1  IntegratorMethod=Forward Euler  FilterMethod=Forward Euler  ControllerParametersSource=internal  P=10  I=0.01  D=0.1  UseFilter=on  N=100  TunerSelectOption=Transfer Function Based (PID Tuner App)  InitialConditionSource=internal  InitialConditionForIntegrator=0  InitialConditionForFilter=0  DifferentiatorICPrevScaledInput=0  ExternalReset=none  TrackingMode=off  Kt=1  LimitOutput=on  SatLimitsSource=internal  UpperSaturationLimit=brakes*Fx_lim*0.25*R - regTorque  LowerSaturationLimit=0  LinearizeAsGain=on  AntiWindupMode=none  Kb=1  POutMin=[]  POutMax=[]  IOutMin=[]  IOutMax=[]  DOutMin=[]  DOutMax=[]  NOutMin=[]  NOutMax=[]  SumOutMin=[]  SumOutMax=[]  SaturationOutMin=[]  SaturationOutMax=[]  PParamMin=[]  PParamMax=[]  IParamMin=[]  IParamMax=[]  DParamMin=[]  DParamMax=[]  NParamMin=[]  NParamMax=[]  KbParamMin=[]  KbParamMax=[]  KtParamMin=[]  KtParamMax=[]  KbOutMin=[]  KbOutMax=[]  KtOutMin=[]  KtOutMax=[]  IntegratorOutMin=[]  IntegratorOutMax=[]  FilterOutMin=[]  FilterOutMax=[]  SumI1OutMin=[]  SumI1OutMax=[]  SumI2OutMin=[]  SumI2OutMax=[]  SumI3OutMin=[]  SumI3OutMax=[]  SumI4OutMin=[]  SumI4OutMax=[]  SumDOutMin=[]  SumDOutMax=[]  DifferentiatorOutMin=[]  DifferentiatorOutMax=[]  FilterDiffOutCoefMin=[]  FilterDiffOutCoefMax=[]  ReciprocalOutMin=[]  ReciprocalOutMax=[]  SumDenOutMin=[]  SumDenOutMax=[]  SumNumOutMin=[]  SumNumOutMax=[]  DivideOutMin=[]  DivideOutMax=[]  UdiffTsProdOutMin=[]  UdiffTsProdOutMax=[]  NTsProdOutMin=[]  NTsProdOutMax=[]  UintegralTsProdOutMin=[]  UintegralTsProdOutMax=[]  UngainTsProdOutMin=[]  UngainTsProdOutMax=[]  IntegratorContinuousStateAttributes=''  IntegratorStateMustResolveToSignalObject=off  IntegratorRTWStateStorageClass=Auto  FilterContinuousStateAttributes=''  FilterStateMustResolveToSignalObject=off  FilterRTWStateStorageClass=Auto  ParallelPVariant=InternalParameters  IdealPVariant=Disabled  IVariant=InternalParameters  DVariant=InternalParameters  IntegratorVariant=Discrete  SatVariant=Enabled  AWVariant=Passthrough  PCopyVariant=Disabled  TRVariant=Disabled  FdbkBlocksVariant=Forward  IdealPFdbkVariant=Disabled  SatFdbkVariant=Disabled  DerivativeFilterVariant=ForwardEulerFilter  NVariant=InternalParameters  NCopyVariant=Disabled  FilterICVariant=InternalICsFilter  IntegratorICVariant=InternalICs  ExternalResetVariant=Disabled  TRSumVariant=Passthrough  SumFdbkVariant=Disabled  SumVariant=Sum_PID  TsampFilterVariant=InternalTs  TsampNgainVariant=Passthrough  TsampIntegralVariant=Passthrough  ExternalSaturationOutDataTypeStr=Inherit: Same as second input
  PID Rear1 : pid_lib/PID Controller  Controller=PID  Form=Parallel  TimeDomain=Discrete-time  UseExternalTs=off  SampleTime=-1  IntegratorMethod=Forward Euler  FilterMethod=Forward Euler  ControllerParametersSource=internal  P=10  I=0.01  D=0.1  UseFilter=on  N=100  TunerSelectOption=Transfer Function Based (PID Tuner App)  InitialConditionSource=internal  InitialConditionForIntegrator=0  InitialConditionForFilter=0  DifferentiatorICPrevScaledInput=0  ExternalReset=none  TrackingMode=off  Kt=1  LimitOutput=on  SatLimitsSource=internal  UpperSaturationLimit=brakes*Fx_lim*0.25*R - regTorque  LowerSaturationLimit=0  LinearizeAsGain=on  AntiWindupMode=none  Kb=1  POutMin=[]  POutMax=[]  IOutMin=[]  IOutMax=[]  DOutMin=[]  DOutMax=[]  NOutMin=[]  NOutMax=[]  SumOutMin=[]  SumOutMax=[]  SaturationOutMin=[]  SaturationOutMax=[]  PParamMin=[]  PParamMax=[]  IParamMin=[]  IParamMax=[]  DParamMin=[]  DParamMax=[]  NParamMin=[]  NParamMax=[]  KbParamMin=[]  KbParamMax=[]  KtParamMin=[]  KtParamMax=[]  KbOutMin=[]  KbOutMax=[]  KtOutMin=[]  KtOutMax=[]  IntegratorOutMin=[]  IntegratorOutMax=[]  FilterOutMin=[]  FilterOutMax=[]  SumI1OutMin=[]  SumI1OutMax=[]  SumI2OutMin=[]  SumI2OutMax=[]  SumI3OutMin=[]  SumI3OutMax=[]  SumI4OutMin=[]  SumI4OutMax=[]  SumDOutMin=[]  SumDOutMax=[]  DifferentiatorOutMin=[]  DifferentiatorOutMax=[]  FilterDiffOutCoefMin=[]  FilterDiffOutCoefMax=[]  ReciprocalOutMin=[]  ReciprocalOutMax=[]  SumDenOutMin=[]  SumDenOutMax=[]  SumNumOutMin=[]  SumNumOutMax=[]  DivideOutMin=[]  DivideOutMax=[]  UdiffTsProdOutMin=[]  UdiffTsProdOutMax=[]  NTsProdOutMin=[]  NTsProdOutMax=[]  UintegralTsProdOutMin=[]  UintegralTsProdOutMax=[]  UngainTsProdOutMin=[]  UngainTsProdOutMax=[]  IntegratorContinuousStateAttributes=''  IntegratorStateMustResolveToSignalObject=off  IntegratorRTWStateStorageClass=Auto  FilterContinuousStateAttributes=''  FilterStateMustResolveToSignalObject=off  FilterRTWStateStorageClass=Auto  ParallelPVariant=InternalParameters  IdealPVariant=Disabled  IVariant=InternalParameters  DVariant=InternalParameters  IntegratorVariant=Discrete  SatVariant=Enabled  AWVariant=Passthrough  PCopyVariant=Disabled  TRVariant=Disabled  FdbkBlocksVariant=Forward  IdealPFdbkVariant=Disabled  SatFdbkVariant=Disabled  DerivativeFilterVariant=ForwardEulerFilter  NVariant=InternalParameters  NCopyVariant=Disabled  FilterICVariant=InternalICsFilter  IntegratorICVariant=InternalICs  ExternalResetVariant=Disabled  TRSumVariant=Passthrough  SumFdbkVariant=Disabled  SumVariant=Sum_PID  TsampFilterVariant=InternalTs  TsampNgainVariant=Passthrough  TsampIntegralVariant=Passthrough  ExternalSaturationOutDataTypeStr=Inherit: Same as second input
  Scope{,1..4,6..12} (12 alike) : Scope
  Scope5 : Scope  NumInputPorts=2
  Sum : Sum  Inputs=|+-
  Switch : Switch  Criteria=u2 > Threshold
  Switch1 : Switch  Criteria=u2 > Threshold
  Output : Outport
  wires:
  v/1 -> EBD/3(v), MATLAB Function2/7(v), MATLAB Function/1(v)
  Mux/1 -> Sum/1
  MATLAB Function/1(req_w) -> Scope6/1, Sum/2
  Sum/1 -> Demux1/1, Scope1/1
  Demux1/1 -> PID Front/1
  Demux1/2 -> PID Rear/1
  PID Rear/1 -> Mux1/2
  PID Front/1 -> Mux1/1
  Mux1/1 -> MATLAB Function2/5(u), Scope/1
  Constant/1 -> MATLAB Function2/1(brakes)
  Constant1/1 -> MATLAB Function2/2(Fx)
  Constant2/1 -> MATLAB Function2/3(ratio)
  Constant3/1 -> MATLAB Function2/4(R)
  MATLAB Function2/3(flag_front) -> ABS active? (front)/1
  ABS active? (front)/1 -> MATLAB Function2/8(flag_f)
  s_front/1 -> Scope3/1, EBD/2(s_f), Mux2/1
  s_rear/1 -> EBD/1(s_r), Mux2/2, Scope4/1
  Mux2/1 -> MATLAB Function2/6(s)
  MATLAB Function2/4(flag_rear) -> ABS active? (rear)/1
  ABS active? (rear)/1 -> MATLAB Function2/9(flag_r)
  w_rear/1 -> Mux/2
  w_front/1 -> Scope2/1, Mux/1
  MATLAB Function2/1(Cf_f) -> Scope5/1, " Lag 2"/1
  MATLAB Function1/1(Cf_r) -> Mux3/2, Scope8/1
  MATLAB Function1/2(Cm) -> Mux3/3, Scope9/1
  Mux3/1 -> Output/1
  " Lag 2"/1 -> Scope5/2, Mux3/1
  Lag 1/1 -> Scope7/1, MATLAB Function1/1(u)
  Constant5/1 -> MATLAB Function1/2(regTorque)
  EBD/1(y) -> Scope12/1, Switch1/2, PID Rear1/1
  Constant6/1 -> Switch1/3, Switch/3
  Switch/1 -> Scope11/1, Min/2
  MATLAB Function2/2(Cf_r) -> Min/1, Scope10/1
  Min/1 -> Lag 1/1
  Constant4/1 -> Switch/2
  Switch1/1 -> Switch/1
  PID Rear1/1 -> Switch1/1

== system model/Tracition Control System/TCS controller ==
  w_rear : Inport
  v : Inport  Port=2
  s_rear : Inport  Port=3
  ABS active? (rear) : Delay  DelayLength=1
  Constant : Constant  Value=pedal
  Constant3 : Constant  Value=R
  Lag 1 : TransferFcn  Denominator=[0.01136 1]
  MATLAB Function : MATLAB Function  TreatAsAtomicUnit=on
  MATLAB Function2 : MATLAB Function  TreatAsAtomicUnit=on
  PID Rear : pid_lib/PID Controller  Controller=PID  Form=Parallel  TimeDomain=Discrete-time  UseExternalTs=off  SampleTime=-1  IntegratorMethod=Forward Euler  FilterMethod=Forward Euler  ControllerParametersSource=internal  P=10  I=0.01  D=0.1  UseFilter=on  N=100  TunerSelectOption=Transfer Function Based (PID Tuner App)  InitialConditionSource=internal  InitialConditionForIntegrator=0  InitialConditionForFilter=0  DifferentiatorICPrevScaledInput=0  ExternalReset=none  TrackingMode=off  Kt=1  LimitOutput=on  SatLimitsSource=internal  UpperSaturationLimit=pedal*Cm  LowerSaturationLimit=0  LinearizeAsGain=on  AntiWindupMode=none  Kb=1  POutMin=[]  POutMax=[]  IOutMin=[]  IOutMax=[]  DOutMin=[]  DOutMax=[]  NOutMin=[]  NOutMax=[]  SumOutMin=[]  SumOutMax=[]  SaturationOutMin=[]  SaturationOutMax=[]  PParamMin=[]  PParamMax=[]  IParamMin=[]  IParamMax=[]  DParamMin=[]  DParamMax=[]  NParamMin=[]  NParamMax=[]  KbParamMin=[]  KbParamMax=[]  KtParamMin=[]  KtParamMax=[]  KbOutMin=[]  KbOutMax=[]  KtOutMin=[]  KtOutMax=[]  IntegratorOutMin=[]  IntegratorOutMax=[]  FilterOutMin=[]  FilterOutMax=[]  SumI1OutMin=[]  SumI1OutMax=[]  SumI2OutMin=[]  SumI2OutMax=[]  SumI3OutMin=[]  SumI3OutMax=[]  SumI4OutMin=[]  SumI4OutMax=[]  SumDOutMin=[]  SumDOutMax=[]  DifferentiatorOutMin=[]  DifferentiatorOutMax=[]  FilterDiffOutCoefMin=[]  FilterDiffOutCoefMax=[]  ReciprocalOutMin=[]  ReciprocalOutMax=[]  SumDenOutMin=[]  SumDenOutMax=[]  SumNumOutMin=[]  SumNumOutMax=[]  DivideOutMin=[]  DivideOutMax=[]  UdiffTsProdOutMin=[]  UdiffTsProdOutMax=[]  NTsProdOutMin=[]  NTsProdOutMax=[]  UintegralTsProdOutMin=[]  UintegralTsProdOutMax=[]  UngainTsProdOutMin=[]  UngainTsProdOutMax=[]  IntegratorContinuousStateAttributes=''  IntegratorStateMustResolveToSignalObject=off  IntegratorRTWStateStorageClass=Auto  FilterContinuousStateAttributes=''  FilterStateMustResolveToSignalObject=off  FilterRTWStateStorageClass=Auto  ParallelPVariant=InternalParameters  IdealPVariant=Disabled  IVariant=InternalParameters  DVariant=InternalParameters  IntegratorVariant=Discrete  SatVariant=Enabled  AWVariant=Passthrough  PCopyVariant=Disabled  TRVariant=Disabled  FdbkBlocksVariant=Forward  IdealPFdbkVariant=Disabled  SatFdbkVariant=Disabled  DerivativeFilterVariant=ForwardEulerFilter  NVariant=InternalParameters  NCopyVariant=Disabled  FilterICVariant=InternalICsFilter  IntegratorICVariant=InternalICs  ExternalResetVariant=Disabled  TRSumVariant=Passthrough  SumFdbkVariant=Disabled  SumVariant=Sum_PID  TsampFilterVariant=InternalTs  TsampNgainVariant=Passthrough  TsampIntegralVariant=Passthrough  ExternalSaturationOutDataTypeStr=Inherit: Same as second input
  Scope : Scope
  Scope1 : Scope
  Scope2 : Scope  NumInputPorts=2
  Scope4 : Scope
  Scope5 : Scope  NumInputPorts=3
  Sum : Sum  Inputs=|+-
  Output : Outport
  wires:
  v/1 -> MATLAB Function/1(v)
  w_rear/1 -> Sum/1
  MATLAB Function/1(req_w) -> Sum/2
  Sum/1 -> PID Rear/1, Scope1/1
  PID Rear/1 -> Scope/1, Scope5/1, MATLAB Function2/3(u)
  Constant/1 -> MATLAB Function2/1(pedal)
  Constant3/1 -> MATLAB Function2/2(R)
  s_rear/1 -> Scope4/1, MATLAB Function2/4(s)
  MATLAB Function2/2(flag_rear) -> ABS active? (rear)/1
  ABS active? (rear)/1 -> MATLAB Function2/5(flag_r)
  MATLAB Function2/1(Cm_tcs) -> Output/1, Scope2/2, Scope5/3, Scope5/2, Scope2/1

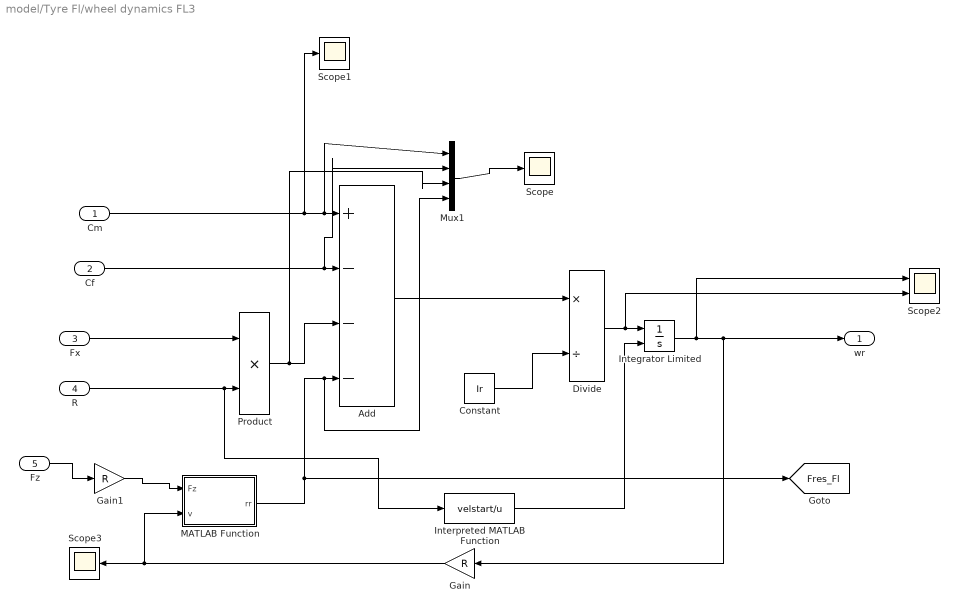
== system model/Tyre Fl/wheel dynamics FL3 ==
  Cm : Inport
  Cf : Inport  Port=2
  Fx : Inport  Port=3
  R : Inport  Port=4
  Fz : Inport  Port=5
  Add : Sum  Inputs=+---
  Constant : Constant  Value=Ir
  Divide : Product  Inputs=*/
  Gain : Gain  Gain=R
  Gain1 : Gain  Gain=R
  Integrator Limited : Integrator  InitialConditionSource=external  LimitOutput=on  LowerSaturationLimit=0
  Interpreted MATLAB Function : MATLABFcn  MATLABFcn=velstart/u
  MATLAB Function : MATLAB Function  TreatAsAtomicUnit=on
  Mux1 : Mux
  Product : Product
  Scope : Scope
  Scope1 : Scope
  Scope2 : Scope  NumInputPorts=2
  Scope3 : Scope
  wr : Outport
  tag scope: Fres_Fl=global
  wires:
  Cm/1 -> Scope1/1, Mux1/1, Add/1
  Divide/1 -> Integrator Limited/1, Scope2/2
  Product/1 -> Mux1/3, Add/3
  R/1 -> Interpreted MATLAB Function/1, Product/2
  Cf/1 -> Mux1/2, Add/2
  Fx/1 -> Product/1
  Constant/1 -> Divide/2
  Mux1/1 -> Scope/1
  Add/1 -> Divide/1
  Interpreted MATLAB Function/1 -> Integrator Limited/2
  Fz/1 -> Gain1/1
  Gain1/1 -> MATLAB Function/1(Fz)
  Integrator Limited/1 -> Scope2/1, wr/1, Gain/1
  Gain/1 -> MATLAB Function/2(v), Scope3/1
  MATLAB Function/1(rr) -> Mux1/4, Add/4, [Fres_Fl]

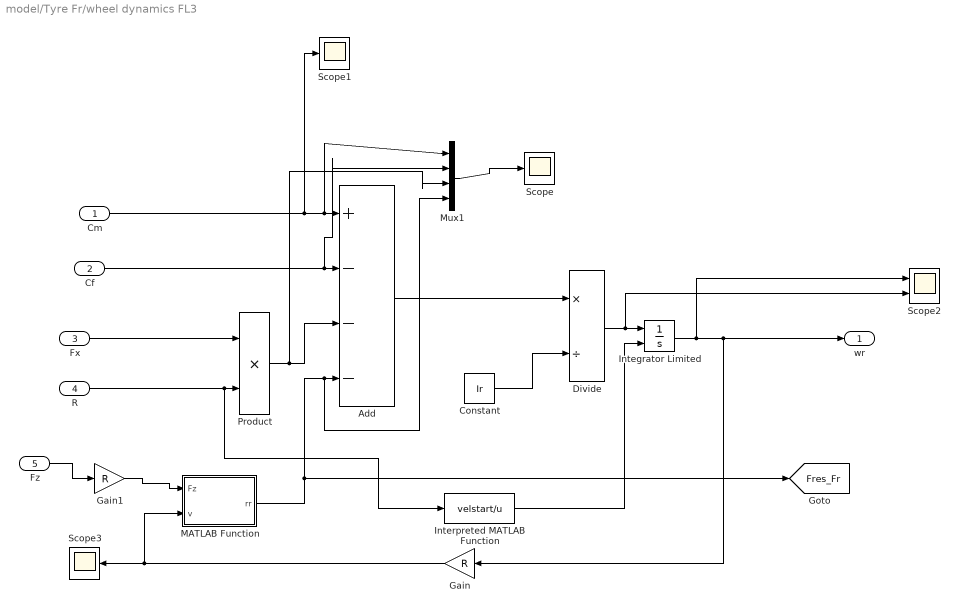
== system model/Tyre Fr/wheel dynamics FL3 ==
  Cm : Inport
  Cf : Inport  Port=2
  Fx : Inport  Port=3
  R : Inport  Port=4
  Fz : Inport  Port=5
  Add : Sum  Inputs=+---
  Constant : Constant  Value=Ir
  Divide : Product  Inputs=*/
  Gain : Gain  Gain=R
  Gain1 : Gain  Gain=R
  Integrator Limited : Integrator  InitialConditionSource=external  LimitOutput=on  LowerSaturationLimit=0
  Interpreted MATLAB Function : MATLABFcn  MATLABFcn=velstart/u
  MATLAB Function : MATLAB Function  TreatAsAtomicUnit=on
  Mux1 : Mux
  Product : Product
  Scope : Scope
  Scope1 : Scope
  Scope2 : Scope  NumInputPorts=2
  Scope3 : Scope
  wr : Outport
  tag scope: Fres_Fr=global
  wires:
  Cm/1 -> Scope1/1, Mux1/1, Add/1
  Divide/1 -> Integrator Limited/1, Scope2/2
  Product/1 -> Mux1/3, Add/3
  R/1 -> Interpreted MATLAB Function/1, Product/2
  Cf/1 -> Mux1/2, Add/2
  Fx/1 -> Product/1
  Constant/1 -> Divide/2
  Mux1/1 -> Scope/1
  Add/1 -> Divide/1
  Interpreted MATLAB Function/1 -> Integrator Limited/2
  Fz/1 -> Gain1/1
  Gain1/1 -> MATLAB Function/1(Fz)
  Integrator Limited/1 -> Scope2/1, wr/1, Gain/1
  Gain/1 -> MATLAB Function/2(v), Scope3/1
  MATLAB Function/1(rr) -> Mux1/4, Add/4, [Fres_Fr]

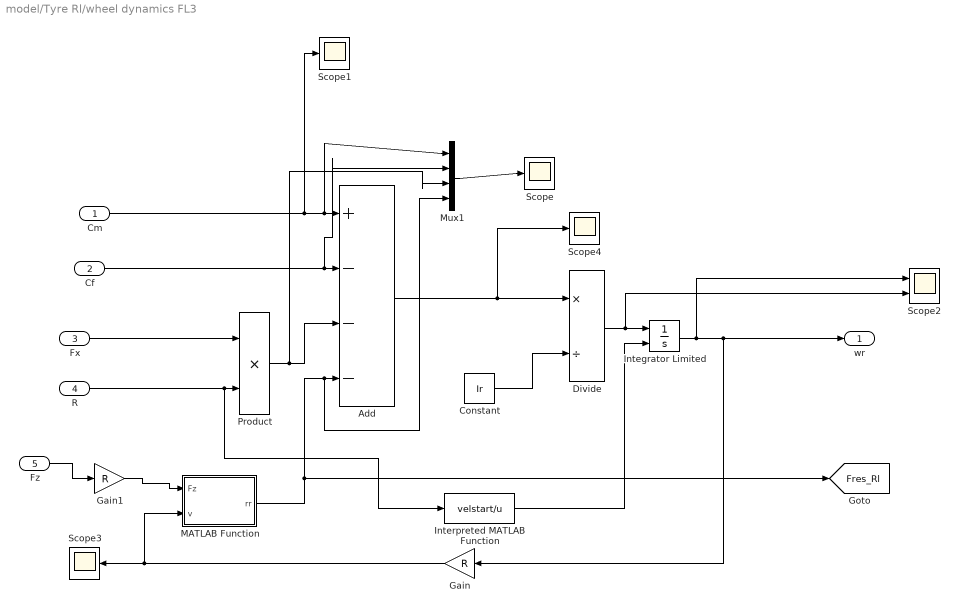
== system model/Tyre Rl/wheel dynamics FL3 ==
  Cm : Inport
  Cf : Inport  Port=2
  Fx : Inport  Port=3
  R : Inport  Port=4
  Fz : Inport  Port=5
  Add : Sum  Inputs=+---
  Constant : Constant  Value=Ir
  Divide : Product  Inputs=*/
  Gain : Gain  Gain=R
  Gain1 : Gain  Gain=R
  Integrator Limited : Integrator  InitialConditionSource=external  LimitOutput=on  LowerSaturationLimit=0
  Interpreted MATLAB Function : MATLABFcn  MATLABFcn=velstart/u
  MATLAB Function : MATLAB Function  TreatAsAtomicUnit=on
  Mux1 : Mux
  Product : Product
  Scope{,1,3..4} (4 alike) : Scope
  Scope2 : Scope  NumInputPorts=2
  wr : Outport
  tag scope: Fres_Rl=global
  wires:
  Cm/1 -> Scope1/1, Mux1/1, Add/1
  Divide/1 -> Integrator Limited/1, Scope2/2
  Product/1 -> Mux1/3, Add/3
  R/1 -> Interpreted MATLAB Function/1, Product/2
  Cf/1 -> Mux1/2, Add/2
  Fx/1 -> Product/1
  Constant/1 -> Divide/2
  Mux1/1 -> Scope/1
  Add/1 -> Scope4/1, Divide/1
  Interpreted MATLAB Function/1 -> Integrator Limited/2
  Fz/1 -> Gain1/1
  Gain1/1 -> MATLAB Function/1(Fz)
  Integrator Limited/1 -> Scope2/1, wr/1, Gain/1
  Gain/1 -> MATLAB Function/2(v), Scope3/1
  MATLAB Function/1(rr) -> Mux1/4, Add/4, [Fres_Rl]

== system model/Tyre Rr/wheel dynamics FL3 ==
  Cm : Inport
  Cf : Inport  Port=2
  Fx : Inport  Port=3
  R : Inport  Port=4
  Fz : Inport  Port=5
  Add : Sum  Inputs=+---
  Constant : Constant  Value=Ir
  Divide : Product  Inputs=*/
  Gain : Gain  Gain=R
  Gain1 : Gain  Gain=R
  Integrator Limited : Integrator  InitialConditionSource=external  LimitOutput=on  LowerSaturationLimit=0
  Interpreted MATLAB Function : MATLABFcn  MATLABFcn=velstart/u
  MATLAB Function : MATLAB Function  TreatAsAtomicUnit=on
  Mux1 : Mux
  Product : Product
  Scope : Scope
  Scope1 : Scope
  Scope2 : Scope  NumInputPorts=2
  Scope3 : Scope
  wr : Outport
  tag scope: Fres_Rr=global
  wires:
  Cm/1 -> Scope1/1, Mux1/1, Add/1
  Divide/1 -> Integrator Limited/1, Scope2/2
  Product/1 -> Mux1/3, Add/3
  R/1 -> Interpreted MATLAB Function/1, Product/2
  Cf/1 -> Mux1/2, Add/2
  Fx/1 -> Product/1
  Constant/1 -> Divide/2
  Mux1/1 -> Scope/1
  Add/1 -> Divide/1
  Interpreted MATLAB Function/1 -> Integrator Limited/2
  Fz/1 -> Gain1/1
  Gain1/1 -> MATLAB Function/1(Fz)
  Integrator Limited/1 -> Scope2/1, wr/1, Gain/1
  Gain/1 -> MATLAB Function/2(v), Scope3/1
  MATLAB Function/1(rr) -> [Fres_Rr], Mux1/4, Add/4

== system model/torque generator/BATTERY ==
  In1 : Inport
  Add : Sum  Inputs=+-
  Constant : Constant  Value=battery_capacity
  Gain : Gain  Gain=100/battery_capacity
  Saturation : Saturate  UpperLimit=battery_capacity  LowerLimit=0
  Scope : Scope
  To Workspace : ToWorkspace  VariableName=battery_charge  SampleTime=-1
  SoC : Outport
  wires:
  Saturation/1 -> To Workspace/1, Gain/1, Scope/1
  Constant/1 -> Add/1
  In1/1 -> Add/2
  Add/1 -> Saturation/1
  Gain/1 -> SoC/1

== matlab function model/Tyre Fl/SLIP RATIO ==
  data: v input; s output; vw input
function s = fcn(v,vw)
    
    s = (vw - v)/v;

== matlab function model/Tyre Fl/wheel dynamics FL3/MATLAB Function ==
  data: Fz input; v input; rr output
function rr = fcn(Fz,v)
    f0 = 0.009;
    f1 = 6.5e-6;
    rr = Fz*(f0 + f1*v^2);
end

== matlab function model/Tyre Fr/Pacejka 1 ==
  settings: fimath=|
      | fimath(...
      | 'RoundMode', 'floor',...
      | 'OverflowMode', 'wrap',...
      | 'ProductMode', 'KeepLSB', 'ProductWordLength', 32,...
      | 'SumMode', 'KeepLSB', 'SumWordLength', 32,...
      | 'CastBeforeSum', false)
  data: Pac input; gamma input; slip input; alfa input; Fz input; F_pac output; mu input; Vcx input; C_F output; R0 input
function [F_pac,C_F] = fcn(Pac,gamma,slip,alfa,Fz,mu,Vcx,R0)
% function for computing forces Fx, Fy and self-aligning torque Mz

% Pac   -> model structure with coeff. Pacejka 96
% slip  -> slip ratio [-] (-1:1)
% alfa  -> slip angle [rad]
% gamma -> camber [rad]
% Vcx,y velocity components of tire contact point C

% Structure building: Pacejka model coefficients
Pa_FZ0_ = Pac(1);
Pa_LFZ0 = Pac(2);
Pa_LmuV = Pac(3);
Pa_LKXK = Pac(4);
Pa_LKYA = Pac(5);
Pa_LCX_ = Pac(6);
Pa_LCY_ = Pac(7);
Pa_LEX_ = Pac(8);
Pa_LEY_ = Pac(9);
Pa_LHX_ = Pac(10);
Pa_LHY_ = Pac(11);
Pa_LVX_ = Pac(12);
Pa_LVY_ = Pac(13);
Pa_LKYG = Pac(14);
Pa_LKZG = Pac(15);
Pa_LT__ = Pac(16);
Pa_MR__ = Pac(17);
Pa_LXA_ = Pac(18);
Pa_LYK_ = Pac(19);
Pa_LVYK = Pac(20);
Pa_LS__ = Pac(21);
Pa_LCZ_ = Pac(22);
Pa_LMX_ = Pac(23);
Pa_LMY_ = Pac(24);
Pa_PCX1 = Pac(25);
Pa_PDX1 = Pac(26);
Pa_PDX2 = Pac(27);
Pa_PEX1 = Pac(28);
Pa_PEX2 = Pac(29);
Pa_PEX3 = Pac(30);
Pa_PEX4 = Pac(31);
Pa_PKX1 = Pac(32);
Pa_PKX2 = Pac(33);
Pa_PKX3 = Pac(34);
Pa_PHX1 = Pac(35);
Pa_PHX2 = Pac(36);
Pa_PVX1 = Pac(37);
Pa_PVX2 = Pac(38);
Pa_RBX1 = Pac(39);
Pa_RBX2 = Pac(40);
Pa_RCX1 = Pac(41);
Pa_RHX1 = Pac(42);
Pa_RTX1 = Pac(43);
Pa_RTX2 = Pac(44);
Pa_RTX3 = Pac(45);
Pa_QSX1 = Pac(46);
Pa_QSX2 = Pac(47);
Pa_QSX3 = Pac(48);
Pa_PCY1 = Pac(49);
Pa_PDY1 = Pac(50);
Pa_PDY2 = Pac(51);
Pa_PDY3 = Pac(52);
Pa_PEY1 = Pac(53);
Pa_PEY2 = Pac(54);
Pa_PEY3 = Pac(55);
Pa_PEY4 = Pac(56);
Pa_PKY1 = Pac(57);
Pa_PKY2 = Pac(58);
Pa_PKY3 = Pac(59);
Pa_PHY1 = Pac(60);
Pa_PHY2 = Pac(61);
Pa_PHY3 = Pac(62);
Pa_PVY1 = Pac(63);
Pa_PVY2 = Pac(64);
Pa_PVY3 = Pac(65);
Pa_PVY4 = Pac(66);
Pa_RBY1 = Pac(67);
Pa_RBY2 = Pac(68);
Pa_RBY3 = Pac(69);
Pa_RCY1 = Pac(70);
Pa_RHY1 = Pac(71);
Pa_RVY1 = Pac(72);
Pa_RVY2 = Pac(73);
Pa_RVY3 = Pac(74);
Pa_RVY4 = Pac(75);
Pa_RVY5 = Pac(76);
Pa_RVY6 = Pac(77);
Pa_PTY1 = Pac(78);
Pa_PTY2 = Pac(79);
Pa_QSY1 = Pac(80);
Pa_QSY2 = Pac(81);
Pa_QBZ1 = Pac(82);
Pa_QBZ2 = Pac(83);
Pa_QBZ3 = Pac(84);
Pa_QBZ4 = Pac(85);
Pa_QBZ5 = Pac(86);
Pa_QBZ6 = Pac(87);
Pa_QBZ9 = Pac(88);
Pa_QBZZ = Pac(89);
Pa_QCZ1 = Pac(90);
Pa_QDZ1 = Pac(91);
Pa_QDZ2 = Pac(92);
Pa_QDZ3 = Pac(93);
Pa_QDZ4 = Pac(94);
Pa_QDZ6 = Pac(95);
Pa_QDZ7 = Pac(96);
Pa_QDZ8 = Pac(97);
Pa_QDZ9 = Pac(98);
Pa_QEZ1 = Pac(99);
Pa_QEZ2 = Pac(100);
Pa_QEZ3 = Pac(101);
Pa_QEZ4 = Pac(102);
Pa_QEZ5 = Pac(103);
Pa_QHZ1 = Pac(104);
Pa_QHZ2 = Pac(105);
Pa_QHZ3 = Pac(106);
Pa_QHZ4 = Pac(107);
Pa_SSZ1 = Pac(108);
Pa_SSZ2 = Pac(109);
Pa_SSZ3 = Pac(110);
Pa_SSZ4 = Pac(111);
Pa_QTZ1 = Pac(112);

% Costants
epsi = 0.01;
eps_V = 0.1;
csi_0=1;
csi_4=1;
Amu = 10;
Pa_LmuX = mu;
Pa_LmuY = mu;

%-------------------------------- Fx pure slip ---------------------------
Cx = Pa_PCX1*Pa_LCX_;
dfz = (Fz-Pa_LFZ0*Pa_FZ0_)/(Pa_LFZ0*Pa_FZ0_);
mux = Pa_LmuX * (Pa_PDX1 + Pa_PDX2 * dfz);
Dx = mux*Fz; %*csi_1, con csi_1=1
%Shx = (Pa_PHX1+Pa_PHX2*dfz)*Pa_LHX_;
Shx = 0;
Kx = slip + Shx;
Ex = (Pa_PEX1+Pa_PEX2*dfz+Pa_PEX3*dfz^2)*(1-Pa_PEX4*sign(Kx))*Pa_LEX_;
if Ex>1 Et=1; end
Kxk = Fz*(Pa_PKX1+Pa_PKX2*dfz)*exp(Pa_PKX3*dfz)*Pa_LKXK;
Bx = Kxk/(Cx*Dx+epsi);
lam_mux  = Pa_LmuX*Amu/(1+(Amu-1)*Pa_LmuX);
SVx = Fz*(Pa_PVX1+Pa_PVX2*dfz)*(abs(Vcx)/(abs(Vcx)+eps_V))*Pa_LVX_*lam_mux; %*csi_1, con csi_1=1

% logitudinal slip stiffness (Fx slope in the origin)
C_Fk = Bx*Cx*Dx;

% longitudinal force
Fx0 = Dx*sin(Cx*atan(Bx*Kx-Ex*(Bx*Kx-atan(Bx*Kx)))) + SVx;

%---------------------------- Fy pure side slip --------------------------
seg=sign(Vcx);
if seg==0 seg=1; end
alfa_star = tan(alfa)*seg;
gam_star = sin(gamma);
Shy = (Pa_PHY1+Pa_PHY2*dfz)*Pa_LHY_+Pa_PHY3*gam_star*Pa_LKYG*csi_0+csi_4-1;
alfa_y = alfa_star + Shy;
Cy = Pa_PCY1*Pa_LCY_;
muy = Pa_LmuY*(Pa_PDY1+Pa_PDY2*dfz)*(1-Pa_PDY3*gam_star^2);
Dy = muy*Fz; %*csi_2, con csi_2=1
Ey = (Pa_PEY1+Pa_PEY2*dfz)*(1-(Pa_PEY3+Pa_PEY4*gam_star)*sign(alfa_y))*Pa_LEY_;
if Ey>1 Ey=1; end
Kya0 = Pa_PKY1*Pa_LFZ0*Pa_FZ0_*sin(2*atan(Fz/(Pa_PKY2*Pa_LFZ0*Pa_FZ0_)))*Pa_LKYA;
Kya = Kya0*(1-Pa_PKY3*gam_star^2); %*csi_3, con csi_3=1
By = Kya/(Cy*Dy+epsi);
lam_muy = Pa_LmuY*Amu/(1+(Amu-1)*Pa_LmuY);
SVy = Fz*((Pa_PVY1+Pa_PVY2*dfz)*Pa_LVY_+(Pa_PVY3+Pa_PVY4*dfz)*gam_star*Pa_LKYG )*lam_muy; %*csi_2, con csi_2=1
Kyg0 = (Pa_PHY3*Kya0+Fz*(Pa_PVY3+Pa_PVY4*dfz))*Pa_LKYG;

% cornering stiffness (Fy slope in the origin)
C_Fa = By*Cy*Dy;

% lateral force
Fy0 = Dy*sin(Cy*atan(By*alfa_y-Ey*(By*alfa_y-atan(By*alfa_y)))) + SVy;

% --------------------- Fx combined slip ------------------------------
Shxa = Pa_RHX1;
%Exa = Pa_REX1+Pa_REX2*dfz; NON esiste Pa.REX1 ne' Pa.REX2
Exa = 0;
Cxa = Pa_RCX1;
Bxa = Pa_RBX1*cos(atan(Pa_RBX2*slip))*Pa_LXA_;
alfaS = alfa_star+Shxa;
Gxa0 = cos(Cxa*atan(Bxa*Shxa-Exa*(Bxa*Shxa-atan(Bxa*Shxa))));
Gxa = cos(Cxa*atan(Bxa*alfaS-Exa*(Bxa*alfaS-atan(Bxa*alfaS))))/Gxa0;
Fx = Fx0*Gxa;

% ---------------------- Fy combined slip ------------------------------
Dvyk = muy*Fz*(Pa_RVY1+Pa_RVY2*dfz+Pa_RVY3*gam_star)*cos(atan(Pa_RVY4*alfa_star));%*csi_2, con csi_2=1
Svyk = Dvyk*sin(Pa_RVY5*atan(Pa_RVY6*slip));
Shyk = Pa_RHY1; %+Pa.RHY2*dfz; NON esiste Pa.RHY2
Cyk = Pa_RCY1;
Byk = Pa_RBY1*cos(atan(Pa_RBY2*(alfa_star-Pa_RBY3)))*Pa_LYK_;
%Eyk = Pa_REY1+Pa_REY2*dfz; NON esiste Pa.REY1 ne' Pa.REY2
Eyk = 0;
ks = slip+Shyk;
Gyk0 = cos(Cyk*atan(Byk*Shyk-Eyk*(Byk*Shyk-atan(Byk*Shyk))));
Gyk = cos(Cyk*atan(Byk*ks-Eyk*(Byk*ks-atan(Byk*ks))))/Gyk0;
Fy = Fy0*Gyk+Svyk;

% --------------------- Mz pure side slip  ---------------------------
Shf = Shy+SVy/Kya;
alfa_r = alfa_star+Shf;
Br = (Pa_QBZ9/Pa_LmuY+Pa_QBZZ*By*Cy); %*csi_6, con csi_6=1
%%% Pa_QBZZ e' in realta' QBZ10 scritto cosi' x ragioni di spazio
Cr = 1; %*csi_7, con csi_7=1
Dr = Fz*R0*((Pa_QDZ6+Pa_QDZ7*dfz)+(Pa_QDZ8+Pa_QDZ9*dfz)*gam_star)*cos(alfa)*Pa_LmuY*seg; %+csi_8-1, con csi_8=1
Mzr0 = Dr*cos(Cr*atan(Br*alfa_r));
Sht = Pa_QHZ1+Pa_QHZ2*dfz+(Pa_QHZ3+Pa_QHZ4*dfz)*gam_star;
alfa_t = alfa_star+Sht;
Bt = (Pa_QBZ1+Pa_QBZ2*dfz+Pa_QBZ3*dfz^2)*(1+Pa_QBZ5*abs(gam_star)+Pa_QBZ6*gam_star^2)*Pa_LKYA/Pa_LmuY;
if Bt<0 Bt=0; end
Ct = Pa_QCZ1;
Dt0 = Fz*R0/(Pa_LFZ0*Pa_FZ0_)*(Pa_QDZ1+Pa_QDZ2*dfz)*seg;
Dt = Dt0*(1+Pa_QDZ3*abs(gam_star)+Pa_QDZ4*gam_star^2); %*csi_5, con csi_5=1
Et = (Pa_QEZ1+Pa_QEZ2*dfz+Pa_QEZ3*dfz^2)*(1+(Pa_QEZ4+Pa_QEZ5*gam_star)*2/pi*atan(Bt*Ct*alfa_t));
if Et>1 Et=1; end
t0 = Dt*cos(Ct*atan(Bt*alfa_t - Et*(Bt*alfa_t-atan(Bt*alfa_t))))*cos(alfa);
Mz0 = -t0*Fy;
Kza0 = Dt0*Kya0;
%Kzg0 = Fz*R0*(Pa_QDZ8+Pa_QDZ9*dfz)-Dt0*Kyg0;

% aligning torque
Mz = Mz0 + Mzr0;

% ------------------------ Mz Combined -----------------------------
eps_k = 0; % 
lambda_s = Pa_LS__ ;
Fz0p = Pa_LFZ0*Pa_FZ0_;
K_yap = Kya + eps_k;
alfa_req = sqrt(alfa_r^2+(Kxk/K_yap)^2*slip^2)*sign(alfa_r);
alfa_teq = sqrt(alfa_t^2+(Kxk/K_yap)^2*slip^2)*sign(alfa_t);
s = R0*(Pa_SSZ1 + Pa_SSZ2*(Fy/Fz0p) + (Pa_SSZ3+Pa_SSZ4*dfz)*gam_star)*lambda_s;
Mzr = Dr*cos(Cr*atan(Br*alfa_req));
Fyp = Fy-Svyk; 
t = Dt*cos(Ct*atan(Bt*alfa_teq - Et*(Bt*alfa_teq-atan(Bt*alfa_teq))))*cos(alfa);
Mzp = -t*Fyp;
% aligning torque
Mz = Mzp + Mzr + s*Fx;
%%%%%%%%%%%%%%%%%%%%%%%

% Check that Fz is positive
if Fz <= 0
    Fx = 0;
    Fy = 0;
    Mz = 0;
end

% Output
F_pac = [Fx; Fy; Mz];
C_F = [C_Fk; C_Fa];

== matlab function model/Tyre Fr/SLIP RATIO ==
  data: v input; s output; vw input
function s = fcn(v,vw)
    
    s = (vw - v)/v;

== matlab function model/Tyre Fr/wheel dynamics FL3/MATLAB Function ==
  data: Fz input; v input; rr output
function rr = fcn(Fz,v)
    f0 = 0.009;
    f1 = 6.5e-6;
    rr = Fz*(f0 + f1*v^2);
end
